simulink model "simulink_02"  (R2014b)
settings: Solver=VariableStepAuto  StartTime=0.0  StopTime=10.0  MaxStep=0.01  RelTol=1e-3
undefined symbols (not defined in the file or in its folder): compv
settings Model: Creator=段润田  LastModifiedBy=treasersmac
settings DataIOCC: LimitDataPoints=off  SaveFormat=Dataset
settings OptimizationCC: UseDivisionForNetSlopeComputation=off  SimCompilerOptimization=off
settings DebuggingCC: SolverPrmCheckMsg=none  FrameProcessingCompatibilityMsg=error
settings HardwareCC: ProdBitPerPointer=64  ProdLargestAtomicFloat=Float  ProdIntDivRoundTo=Zero  ProdEndianess=LittleEndian  ProdWordSize=64  ProdHWDeviceType=Intel->x86-64 (Windows64)
settings ModelReferenceCC: PropagateSignalLabelsOutOfModel=on
settings RTWCC: RTWCompilerOptimization=off
settings ConfigComp: CovMetricSettings=dw  CovHtmlReporting=on  CovSaveCumulativeToWorkspaceVar=on  CovSaveSingleToWorkspaceVar=on  CovExternalEMLEnable=off

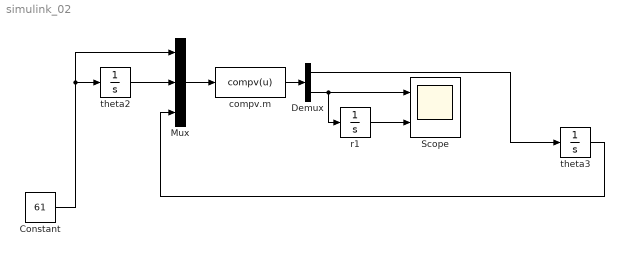
== system simulink_02 ==
  Constant : Constant  Value=61
  Demux : Demux  Outputs=2
  Mux : Mux  Inputs=3
  Scope : Scope  NumInputPorts=2
      settings: YMin=-116.628~-5  YMax=116.628~5
  compv.m : MATLABFcn  MATLABFcn=compv(u)
  r1 : Integrator
  theta2 : Integrator
  theta3 : Integrator
  wires:
  Constant/1 -> Mux/1, theta2/1
  theta2/1 -> Mux/2
  Demux/1 -> theta3/1
  r1/1 -> Scope/2
  Demux/2 -> r1/1, Scope/1
  theta3/1 -> Mux/3
  Mux/1 -> compv.m/1
  compv.m/1 -> Demux/1
